simulink model "version1"  (R2022a)
settings: Solver=VariableStepAuto  StartTime=0.0  StopTime=10.0  RelTol=1e-3
settings Model: Creator=THIS PC  LastModifiedBy=THIS PC

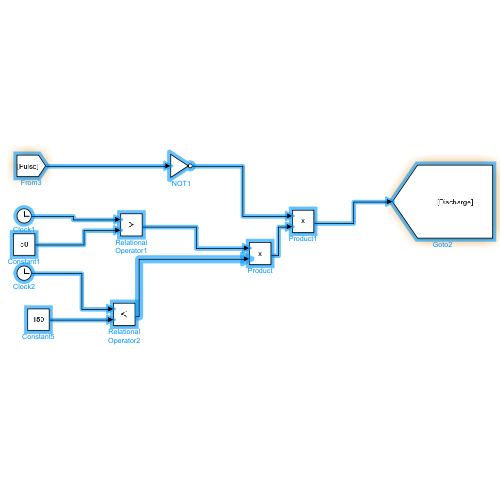
[thumbnail: Simulink's stored preview of the top-level diagram]
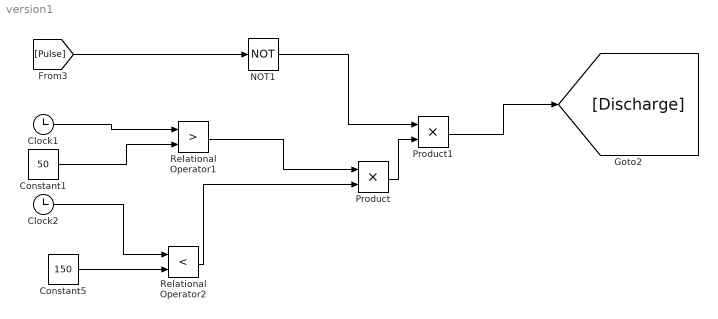
== system version1 ==
  Clock1 : Clock
  Clock2 : Clock
  Constant1 : Constant  Value=50
  Constant5 : Constant  Value=150
  NOT1 : Logic  Operator=NOT  IconShape=distinctive  AllPortsSameDT=off  OutDataTypeStr=boolean
  Product : Product
  Product1 : Product
  Relational Operator1 : RelationalOperator  Operator=>  OutDataTypeStr=boolean  RndMeth=Simplest  InputSameDT=off
  Relational Operator2 : RelationalOperator  Operator=<  OutDataTypeStr=boolean  RndMeth=Simplest  InputSameDT=off
  wires:
  Relational Operator1/1 -> Product/1
  Clock2/1 -> Relational Operator2/1
  Product1/1 -> [Discharge]
  [Pulse] -> NOT1/1
  Constant5/1 -> Relational Operator2/2
  Product/1 -> Product1/2
  Constant1/1 -> Relational Operator1/2
  Clock1/1 -> Relational Operator1/1
  NOT1/1 -> Product1/1
  Relational Operator2/1 -> Product/2
